simulink model "the_last_domaci"  (R2016a)
settings: Solver=VariableStepAuto  StartTime=0.0  StopTime=10  RelTol=1e-3
values from neighbouring files (symbols this model uses):
  A = [1 a 0]    [main.m]
  Am = [1 alpha1 alpha0]    [main.m]
  B = [b]    [main.m]
  Bm = [alpha0]    [main.m]
  R = [1 r0]    [main.m]
  S = [p1 p0]    [main.m]
  T = [t1 t0]    [main.m]
settings Model: Creator=Vukan  LastModifiedBy=Vukan

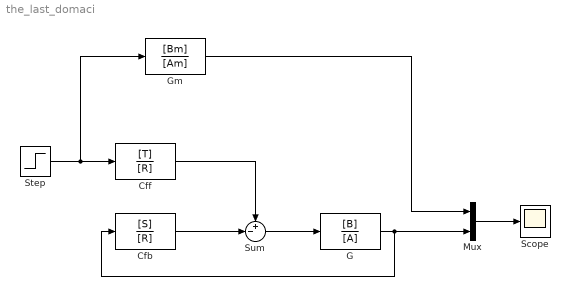
== system the_last_domaci ==
  Cfb : TransferFcn  Numerator=[S]  Denominator=[R]
  Cff : TransferFcn  Numerator=[T]  Denominator=[R]
  G : TransferFcn  Numerator=[B]  Denominator=[A]
  Gm : TransferFcn  Numerator=[Bm]  Denominator=[Am]
  Mux : Mux  Inputs=2
  Scope : Scope
  Step : Step  SampleTime=0
  Sum : Sum  Inputs=+-|
  wires:
  Cfb/1 -> Sum/2
  Cff/1 -> Sum/1
  Sum/1 -> G/1
  G/1 -> Mux/2, Cfb/1
  Step/1 -> Gm/1, Cff/1
  Mux/1 -> Scope/1
  Gm/1 -> Mux/1
